simulink model "FFT4dSpace_rtKolloq_1"  (R2021a)
settings: Solver=FixedStepDiscrete  StartTime=0.0  StopTime=10  FixedStep=1e-5 % Ts  RelTol=1e-3
values from neighbouring files (symbols this model uses):
  NFFT2 = 2^10    (= 1024)    [FFT4dSpace_rtKolloq_1_i.m]    (also in FFT4dSpace_rtKolloq_i.m)
  Ts = 1e-3    (= 0.001)    [FFT4dSpace_rtKolloq_1_i.m]    (also in FFT4dSpace_rtKolloq_i.m)
undefined symbols (not defined in the file or in its folder): mdlPara
libraries: dspxfrm3 x1
settings Model: Creator=nitr  LastModifiedBy=nitr

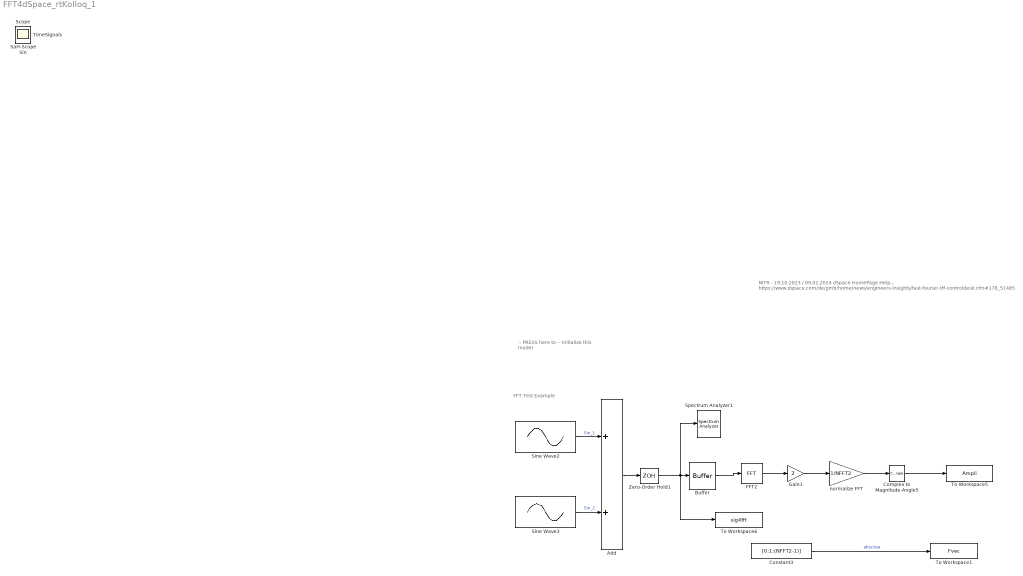
== system FFT4dSpace_rtKolloq_1 ==
  note: NITR - 19.10.2023 / 09.02.2024
      |
      | dSpace HomePage Help...
      | https://www.dspace.com/de/gmb/home/news/engineers-insights/fast-fourier-ttf-controldesk.cfm#178_51485
  note: -- PRESS here to --
      | Initialize this model
  note: FFT Test Example
  Add : Sum
  Buffer : Buffer  N=NFFT2  OutputFrames=off
  Complex to Magnitude-Angle5 : ComplexToMagnitudeAngle  Output=Magnitude
  Constant3 : Constant  Value=[0:1:(NFFT2-1)]
  FFT2 : dspxfrm3/FFT  FFTImplementation=Auto  CompMethod=Table lookup  TableOpt=NEW  TableOptActive=Speed  BitRevOrder=off  Normalize=off  InheritFFTLength=off  FFTLength=NFFT2  WrapInput=on  roundingMode=Floor  overflowMode=off  firstCoeffDataTypeStr=Inherit: Same word length as input  firstCoeffLastDataTypeStr=Inherit: Same word length as input  outputMin=[]  outputMax=[]
  Gain1 : Gain  Gain=2
  Sine Wave2 : Sin  Amplitude=mdlPara.a1  Bias=mdlPara.Bias1  Frequency=mdlPara.om1  SampleTime=0
  Sine Wave3 : Sin  Amplitude=mdlPara.a2  Bias=mdlPara.Bias2  Frequency=mdlPara.om2  SampleTime=0
  Spectrum Analyzer1 : SpectrumAnalyzer
  To Workspace1 : ToWorkspace  VariableName=Fvec  SampleTime=-1
  To Workspace5 : ToWorkspace  VariableName=Ampli  SampleTime=-1
  To Workspace6 : ToWorkspace  VariableName=sig4fft  SaveFormat=Structure With Time  SampleTime=Ts
  Zero-Order Hold1 : ZeroOrderHold  SampleTime=Ts
  normalize FFT : Gain  Gain=1/NFFT2
  SaH-Scope : Scope
  Scope : Scope
  Sin : Scope
  TimeSignals : Scope
  wires:
  Constant3/1 -> To Workspace1/1  "abscissa"
  Buffer/1 -> FFT2/1
  Gain1/1 -> normalize FFT/1
  Sine Wave3/1 -> Add/2  "Sin_2"
  Sine Wave2/1 -> Add/1  "Sin_1"
  Add/1 -> Zero-Order Hold1/1
  normalize FFT/1 -> Complex to Magnitude-Angle5/1
  FFT2/1 -> Gain1/1
  Complex to Magnitude-Angle5/1 -> To Workspace5/1
  Zero-Order Hold1/1 -> Buffer/1, Spectrum Analyzer1/1, To Workspace6/1
